simulink model "ESO"  (Simulink 8.3)
settings: Solver=ode3  StartTime=0.0  StopTime=100  FixedStep=0.001  RelTol=1e-3
values from neighbouring files (symbols this model uses):
  A2 = [0,-1.15000000000000,0,0,0,0,0,0,0,0,0,0,0;0,0.800000000000000,0,0,0,0,0,0,0,9.12000000000000,-1.16000000000000,15.2700000000000,0;0,0,-0.800000000000000,0,0,0,0,0,0,-1.16000000000000,-9.12000000000000,0,-15.2700000000000;0,0,-1.23000000000000,0,0,0,0,0,0,-1,0,0,0;0,0,0,0,0,0,0,0,0,0,-1,0,0;0,0,-1.15000000000000,9,0,0,0,-1,0,-1.50000000000000,-150,1.75000000000000,0;0,0,0,0,9,0,0,0,-1,150,-1.50000 ...(+638 chars)    [ISF1.m]    (also in SF_2.m; ga.m; mycostsmc.m)
  Abar = [A2,zeros(13,13);zeros(13,26)]    [ga.m]
  B2 = [0,0,-1;0,0,0;0,0,0;0,0,0;0,0,0;0,0,0;0,0,0;0,0,0;0,0,0;0,0,0;0,0,0;-2.85713770000155,-0.00542856816238154,0;0.00542856816238154,-2.85713770000155,0]    [ISF1.m]    (also in SF_2.m; ga.m; mycostsmc.m)
  Bbar = [B2;zeros(13,3)]    [ga.m]
  C2 = [0,-0.000150000000000000,0,0,0,0,0,0,0,0,0,0,0;1.42833739578288,0,0,0,0,0,0,0,0,0,0,0.999998195000543,-0.00189999885683354;11.4027344213486,0,0,0,0,0,0,0,0,0,0,0.00189999885683354,0.999998195000543]    [ISF1.m]    (also in SF_2.m; ga.m)
  Cbar = [C2,zeros(3,13)]    [ga.m]
  Kg = -inv(C2*(Am\B2))    [ga.m]
  Km = [K(1,1:13);K(2,1:13);K(3,1:13)]    [ga.m]
  L = ones(26,3)    [ga.m]
  N = zeros(13,13)    [ga.m]
settings Model: Creator=Toshani  LastModifiedBy=Toshani
settings DataIOCC: SignalLoggingSaveFormat=Dataset
settings DebuggingCC: UnderspecifiedInitializationDetection=Simplified  StateNameClashWarn=none
settings GRTTargetCC: CombineOutputUpdateFcns=on  GRTInterface=off

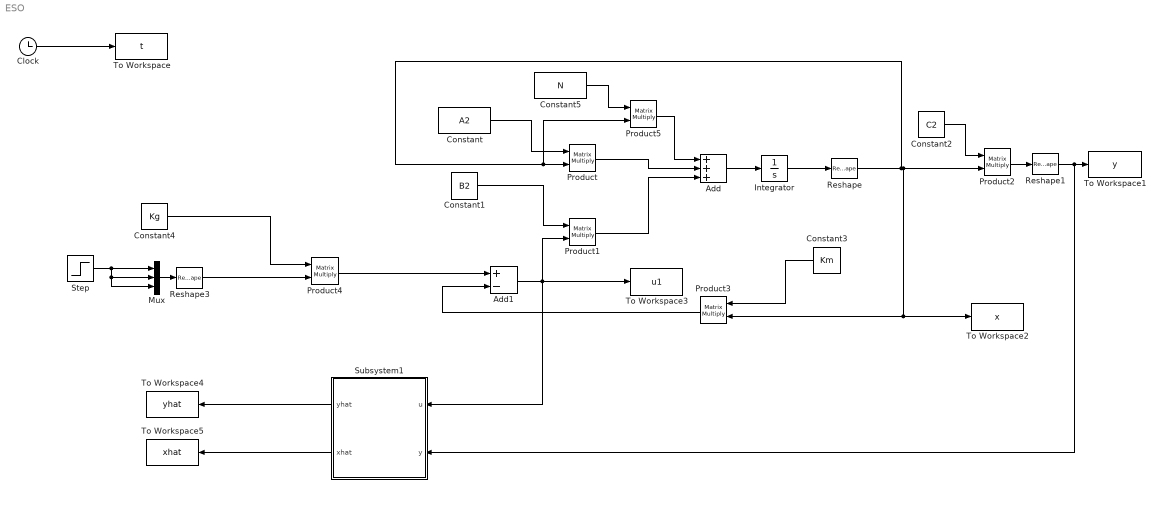
== system ESO ==
  Add : Sum  Inputs=+++
  Add1 : Sum  Inputs=+-
  Clock : Clock
  Constant : Constant  Value=A2
  Constant1 : Constant  Value=B2
  Constant2 : Constant  Value=C2
  Constant3 : Constant  Value=Km
  Constant4 : Constant  Value=Kg
  Constant5 : Constant  Value=N
  Integrator : Integrator  InitialCondition=0.1
  Mux : Mux  Inputs=3
  Product{,1..5} (6 alike) : Product  Multiplication=Matrix(*)
  Reshape : Reshape  OutputDimensionality=Column vector (2-D)
  Reshape1 : Reshape  OutputDimensionality=Column vector (2-D)
  Reshape3 : Reshape  OutputDimensionality=Column vector (2-D)
  Step : Step  Time=0  SampleTime=0
  Subsystem1 : Subsystem
  To Workspace : ToWorkspace  VariableName=t  SampleTime=-1
  To Workspace1 : ToWorkspace  VariableName=y  SampleTime=-1
  To Workspace2 : ToWorkspace  VariableName=x  SampleTime=-1
  To Workspace3 : ToWorkspace  VariableName=u1  SampleTime=-1
  To Workspace4 : ToWorkspace  VariableName=yhat  SampleTime=-1
  To Workspace5 : ToWorkspace  VariableName=xhat  SampleTime=-1
  wires:
  Constant/1 -> Product/1
  Constant1/1 -> Product1/1
  Add/1 -> Integrator/1
  Integrator/1 -> Reshape/1
  Mux/1 -> Reshape3/1
  Step/1 -> Mux/3, Mux/2, Mux/1
  Reshape/1 -> Product3/2, To Workspace2/1, Product2/2, Product5/2, Product/2
  Clock/1 -> To Workspace/1
  Product2/1 -> Reshape1/1
  Constant3/1 -> Product3/1
  Constant2/1 -> Product2/1
  Reshape1/1 -> Subsystem1/2(y), To Workspace1/1
  Reshape3/1 -> Product4/2
  Constant4/1 -> Product4/1
  Product3/1 -> Add1/2
  Product4/1 -> Add1/1
  Add1/1 -> Subsystem1/1(u), To Workspace3/1, Product1/2
  Subsystem1/1(yhat) -> To Workspace4/1
  Subsystem1/2(xhat) -> To Workspace5/1
  Product1/1 -> Add/3
  Product/1 -> Add/2
  Product5/1 -> Add/1
  Constant5/1 -> Product5/1

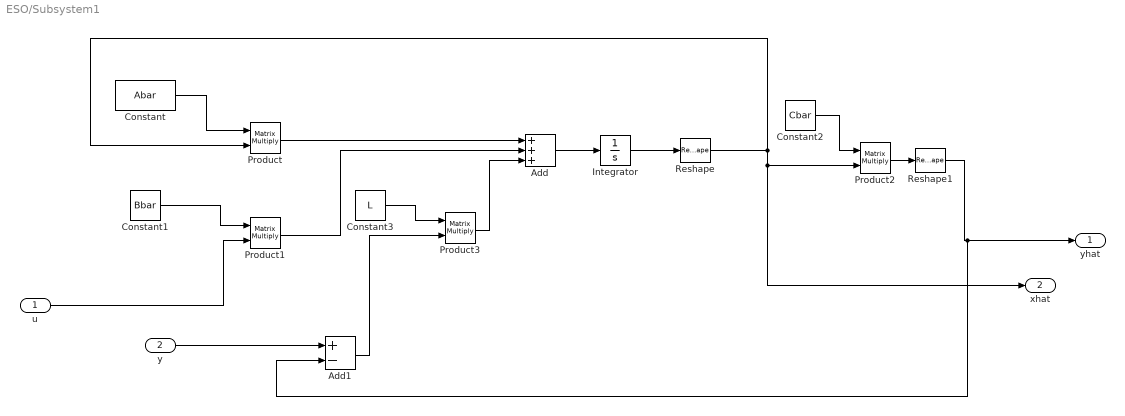
== system ESO/Subsystem1 ==
  u : Inport
  y : Inport  Port=2
  Add : Sum  Inputs=+++
  Add1 : Sum  Inputs=+-
  Constant : Constant  Value=Abar
  Constant1 : Constant  Value=Bbar
  Constant2 : Constant  Value=Cbar
  Constant3 : Constant  Value=L
  Integrator : Integrator  InitialCondition=0.1
  Product{,1..3} (4 alike) : Product  Multiplication=Matrix(*)
  Reshape : Reshape  OutputDimensionality=Column vector (2-D)
  Reshape1 : Reshape  OutputDimensionality=Column vector (2-D)
  yhat : Outport
  xhat : Outport  Port=2
  wires:
  u/1 -> Product1/2
  Reshape1/1 -> Add1/2, yhat/1
  Constant2/1 -> Product2/1
  Product2/1 -> Reshape1/1
  Reshape/1 -> Product2/2, xhat/1, Product/2
  Integrator/1 -> Reshape/1
  Add/1 -> Integrator/1
  Product1/1 -> Add/2
  Constant1/1 -> Product1/1
  Product/1 -> Add/1
  Constant/1 -> Product/1
  y/1 -> Add1/1
  Add1/1 -> Product3/2
  Product3/1 -> Add/3
  Constant3/1 -> Product3/1
